simulink model "logistic_eq_delay"  (R2022a)
settings: Solver=VariableStepAuto  StartTime=0.0  StopTime=40  RelTol=1e-3
settings Model: Creator=Home computer  LastModifiedBy=Home computer

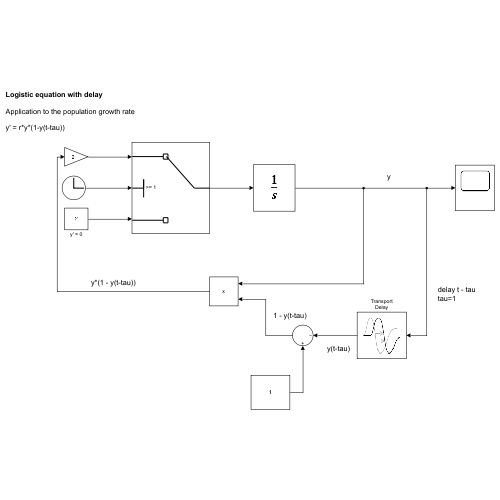
[thumbnail: Simulink's stored preview of the top-level diagram]
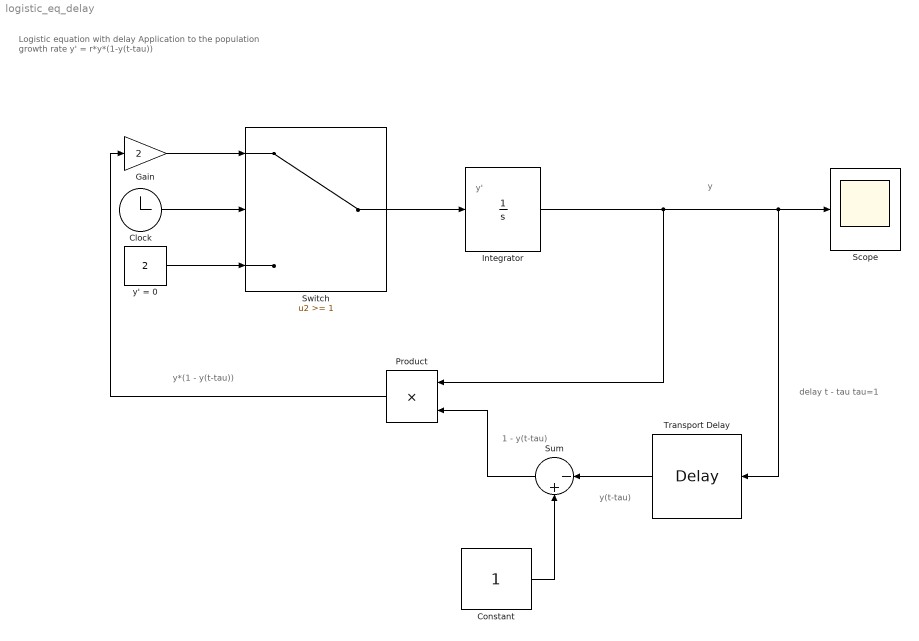
== system logistic_eq_delay ==
  note: Logistic equation with delay
      |
      | Application to the population growth rate
      |
      | y' = r*y*(1-y(t-tau))
  note: y*(1 - y(t-tau))
  note: y(t-tau)
  note: 1 - y(t-tau)
  note: delay t - tau
      | tau=1
  note: y
  note: y'
  Clock : Clock
  Constant : Constant
  Gain : Gain  Gain=2
  Integrator : Integrator
  Product : Product
  Scope : Scope
  Sum : Sum  Inputs=|-+
  Switch : Switch  Threshold=1  SaturateOnIntegerOverflow=off  InputSameDT=off
  Transport Delay : TransportDelay
  y' = 0 : Constant  Value=2
  wires:
  Switch/1 -> Integrator/1
  Integrator/1 -> Scope/1, Transport Delay/1, Product/1
  Clock/1 -> Switch/2
  y' = 0/1 -> Switch/3
  Gain/1 -> Switch/1
  Constant/1 -> Sum/2
  Transport Delay/1 -> Sum/1
  Sum/1 -> Product/2
  Product/1 -> Gain/1
